simulink model "FlightGearScreen"  (R2020b)
settings: Solver=VariableStepAuto  StartTime=0.0  StopTime=10  RelTol=1e-3
values from neighbouring files (symbols this model uses):
  A = [-0.0558 -0.9968 0.0802 0.0415; 0.5980 -0.1150 -0.0318 0; -3.0500 0.3880 -0.4650 0; 0 0.0805 1 0]    [AircraftPaper.m]
  B = [0.0729 0; -4.7500 0.00775; 0.153 0.143; 0 0]    [AircraftPaper.m]
  C = [1 0 0 0; 0 0 0 1]    [AircraftPaper.m]
  Kc = lqr(A,B,Q,R)    [AircraftPaper.m]
  x0 = [pi/6 0 0 pi/4]    [AircraftPaper.m]
libraries: aerolibutil x2, aerolibconvert2 x1, vrlib x1
settings Model: Creator=leobartowski  LastModifiedBy=leobartowski

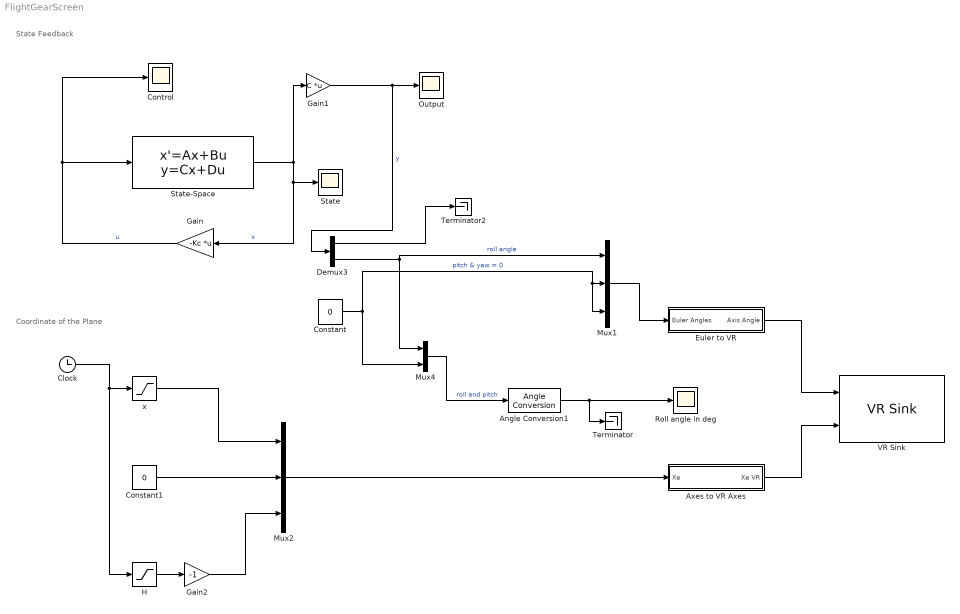
== system FlightGearScreen ==
  note: Coordinate of the Plane
  note: State Feedback
  Angle Conversion1 : aerolibconvert2/Angle Conversion  IU=rad  OU=deg
  Axes to VR Axes : Subsystem
  Clock : Clock
  Constant : Constant  Value=0
  Constant1 : Constant  Value=0
  Control : Scope
  Demux3 : Demux  Outputs=2
  Euler to VR : Subsystem
  Gain : Gain  Gain=-Kc  Multiplication=Matrix(K*u)
  Gain1 : Gain  Gain=C  Multiplication=Matrix(K*u)
  Gain2 : Gain  Gain=-1
  H : Saturate
  Mux1 : Mux  Inputs=3
  Mux2 : Mux  Inputs=3
  Mux4 : Mux  Inputs=2
  Output : Scope
  Roll angle in deg : Scope
  State : Scope
  State-Space : StateSpace  A=A  B=B  C=eye(4)  D=zeros(4,2)  InitialCondition=x0
  Terminator : Terminator
  Terminator2 : Terminator
  VR Sink : vrlib/VR Sink  InstantiateOnLoad=on  SampleTime=0.01  ViewEnable=on  RemoteChange=off  RemoteView=off  FieldsWritten=HL20.rotation.4.1.1.double#HL20.translation.3.1.1.double  WorldFileName=world2.wrl  WorldDescription=Esame MFC  AutoView=on  VideoDimensions=[]  AllowVariableSize=off
  x : Saturate
  wires:
  Euler to VR/1(Axis Angle) -> VR Sink/1
  Axes to VR Axes/1(Xe VR) -> VR Sink/2
  Clock/1 -> H/1, x/1
  x/1 -> Mux2/1
  Constant1/1 -> Mux2/2
  H/1 -> Gain2/1
  Gain2/1 -> Mux2/3
  Mux2/1 -> Axes to VR Axes/1(Xe)
  Constant/1 -> Mux4/2, Mux1/3, Mux1/2  "pitch & yaw = 0"
  Mux1/1 -> Euler to VR/1(Euler Angles)
  State-Space/1 -> Gain1/1, Gain/1, State/1  "x"
  Gain/1 -> Control/1, State-Space/1  "u"
  Gain1/1 -> Demux3/1, Output/1  "y"
  Demux3/1 -> Terminator2/1
  Demux3/2 -> Mux1/1, Mux4/1  "roll angle"
  Mux4/1 -> Angle Conversion1/1  "roll and pitch"
  Angle Conversion1/1 -> Roll angle in deg/1, Terminator/1

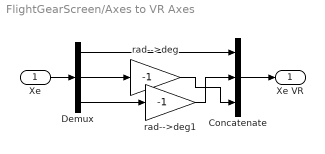
== system FlightGearScreen/Axes to VR Axes ==
  Xe : Inport
  Concatenate : Concatenate  NumInputs=3
  Demux : Demux  Outputs=3
      settings: DisplayOption=none
  rad-->deg : Gain  Gain=-1  SaturateOnIntegerOverflow=on  OutDataTypeStr=Inherit: Same as input  ParamDataTypeStr=Inherit: Same as input
  rad-->deg1 : Gain  Gain=-1  SaturateOnIntegerOverflow=on  OutDataTypeStr=Inherit: Same as input  ParamDataTypeStr=Inherit: Same as input
  Xe VR : Outport  VectorParamsAs1DForOutWhenUnconnected=off
  wires:
  Xe/1 -> Demux/1
  Demux/1 -> Concatenate/1
  Demux/2 -> rad-->deg/1
  Demux/3 -> rad-->deg1/1
  Concatenate/1 -> Xe VR/1
  rad-->deg1/1 -> Concatenate/2
  rad-->deg/1 -> Concatenate/3

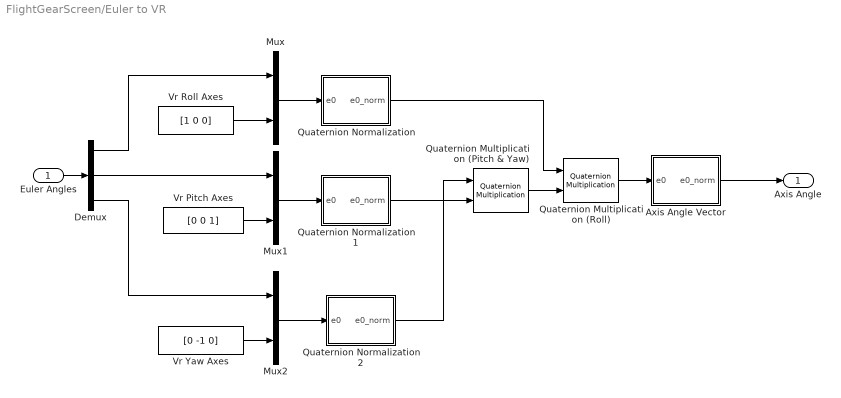
== system FlightGearScreen/Euler to VR ==
  Euler Angles : Inport
  Axis Angle Vector : Subsystem
  Demux : Demux  Outputs=3
      settings: DisplayOption=none
  Mux : Mux  Inputs=2
  Mux1 : Mux  Inputs=2
  Mux2 : Mux  Inputs=2
  Quaternion Multiplication (Pitch & Yaw) : aerolibutil/Quaternion Multiplication
  Quaternion Multiplication (Roll) : aerolibutil/Quaternion Multiplication
  Quaternion Normalization : Subsystem
  Quaternion Normalization1 : Subsystem
  Quaternion Normalization2 : Subsystem
  Vr Pitch Axes : Constant  Value=[0 0 1]
  Vr Roll Axes : Constant  Value=[1 0 0]
  Vr Yaw Axes : Constant  Value=[0 -1 0]
  Axis Angle : Outport  VectorParamsAs1DForOutWhenUnconnected=off
  wires:
  Quaternion Multiplication (Roll)/1 -> Axis Angle Vector/1(e0)
  Quaternion Multiplication (Pitch & Yaw)/1 -> Quaternion Multiplication (Roll)/2
  Axis Angle Vector/1(e0_norm) -> Axis Angle/1
  Quaternion Normalization/1(e0_norm) -> Quaternion Multiplication (Roll)/1
  Quaternion Normalization2/1(e0_norm) -> Quaternion Multiplication (Pitch & Yaw)/1
  Quaternion Normalization1/1(e0_norm) -> Quaternion Multiplication (Pitch & Yaw)/2
  Mux2/1 -> Quaternion Normalization2/1(e0)
  Mux1/1 -> Quaternion Normalization1/1(e0)
  Mux/1 -> Quaternion Normalization/1(e0)
  Demux/3 -> Mux2/1
  Vr Yaw Axes/1 -> Mux2/2
  Demux/2 -> Mux1/1
  Vr Pitch Axes/1 -> Mux1/2
  Demux/1 -> Mux/1
  Vr Roll Axes/1 -> Mux/2
  Euler Angles/1 -> Demux/1

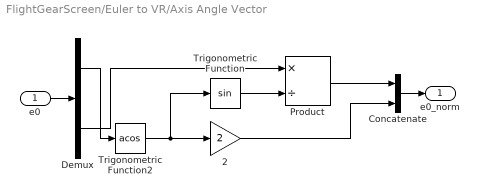
== system FlightGearScreen/Euler to VR/Axis Angle Vector ==
  e0 : Inport
  2 : Gain  Gain=2  SaturateOnIntegerOverflow=on  OutDataTypeStr=Inherit: Same as input  ParamDataTypeStr=Inherit: Same as input
  Concatenate : Concatenate
  Demux : Demux  Outputs=[1 3 ]
      settings: DisplayOption=none
  Product : Product  Inputs=*/  InputSameDT=on  SaturateOnIntegerOverflow=on  OutDataTypeStr=Inherit: Same as first input
  Trigonometric Function : Trigonometry
  Trigonometric Function2 : Trigonometry  Operator=acos
  e0_norm : Outport  VectorParamsAs1DForOutWhenUnconnected=off
  wires:
  Demux/1 -> Trigonometric Function2/1
  Demux/2 -> Product/1
  Concatenate/1 -> e0_norm/1
  Product/1 -> Concatenate/1
  2/1 -> Concatenate/2
  Trigonometric Function/1 -> Product/2
  Trigonometric Function2/1 -> Trigonometric Function/1, 2/1
  e0/1 -> Demux/1

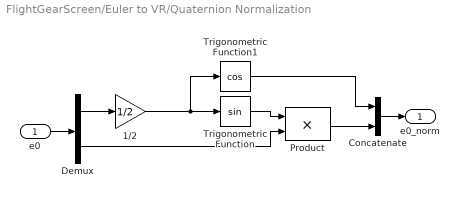
== system FlightGearScreen/Euler to VR/Quaternion Normalization ==
  e0 : Inport
  1/2 : Gain  Gain=1/2  SaturateOnIntegerOverflow=on  OutDataTypeStr=Inherit: Same as input  ParamDataTypeStr=Inherit: Same as input
  Concatenate : Concatenate
  Demux : Demux  Outputs=[1 3]
      settings: DisplayOption=none
  Product : Product  InputSameDT=on  SaturateOnIntegerOverflow=on  OutDataTypeStr=Inherit: Same as first input
  Trigonometric Function : Trigonometry
  Trigonometric Function1 : Trigonometry  Operator=cos
  e0_norm : Outport  VectorParamsAs1DForOutWhenUnconnected=off
  wires:
  Trigonometric Function1/1 -> Concatenate/1
  Demux/2 -> Product/2
  Demux/1 -> 1/2/1
  Concatenate/1 -> e0_norm/1
  Product/1 -> Concatenate/2
  Trigonometric Function/1 -> Product/1
  1/2/1 -> Trigonometric Function1/1, Trigonometric Function/1
  e0/1 -> Demux/1

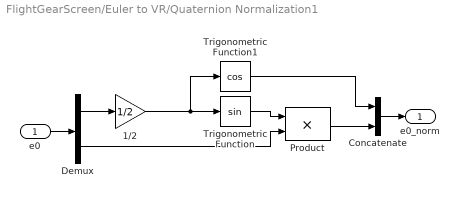
== system FlightGearScreen/Euler to VR/Quaternion Normalization1 ==
  e0 : Inport
  1/2 : Gain  Gain=1/2  SaturateOnIntegerOverflow=on  OutDataTypeStr=Inherit: Same as input  ParamDataTypeStr=Inherit: Same as input
  Concatenate : Concatenate
  Demux : Demux  Outputs=[1 3]
      settings: DisplayOption=none
  Product : Product  InputSameDT=on  SaturateOnIntegerOverflow=on  OutDataTypeStr=Inherit: Same as first input
  Trigonometric Function : Trigonometry
  Trigonometric Function1 : Trigonometry  Operator=cos
  e0_norm : Outport  VectorParamsAs1DForOutWhenUnconnected=off
  wires:
  e0/1 -> Demux/1
  1/2/1 -> Trigonometric Function/1, Trigonometric Function1/1
  Trigonometric Function/1 -> Product/1
  Product/1 -> Concatenate/2
  Concatenate/1 -> e0_norm/1
  Demux/1 -> 1/2/1
  Demux/2 -> Product/2
  Trigonometric Function1/1 -> Concatenate/1

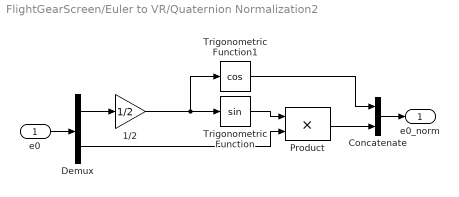
== system FlightGearScreen/Euler to VR/Quaternion Normalization2 ==
  e0 : Inport
  1/2 : Gain  Gain=1/2  SaturateOnIntegerOverflow=on  OutDataTypeStr=Inherit: Same as input  ParamDataTypeStr=Inherit: Same as input
  Concatenate : Concatenate
  Demux : Demux  Outputs=[1 3]
      settings: DisplayOption=none
  Product : Product  InputSameDT=on  SaturateOnIntegerOverflow=on  OutDataTypeStr=Inherit: Same as first input
  Trigonometric Function : Trigonometry
  Trigonometric Function1 : Trigonometry  Operator=cos
  e0_norm : Outport  VectorParamsAs1DForOutWhenUnconnected=off
  wires:
  Trigonometric Function1/1 -> Concatenate/1
  Demux/2 -> Product/2
  Demux/1 -> 1/2/1
  Concatenate/1 -> e0_norm/1
  Product/1 -> Concatenate/2
  Trigonometric Function/1 -> Product/1
  1/2/1 -> Trigonometric Function1/1, Trigonometric Function/1
  e0/1 -> Demux/1
